simulink model "DC_Motor_Modelling"  (R2022b)
settings: Solver=VariableStepAuto  StartTime=0.0  StopTime=100.0  RelTol=1e-3
undefined symbols (not defined in the file): J, Kb, Ktq, L, plecs, R
libraries: ee_lib x3, fl_lib x1
settings Model: Creator=tedro  LastModifiedBy=tedro

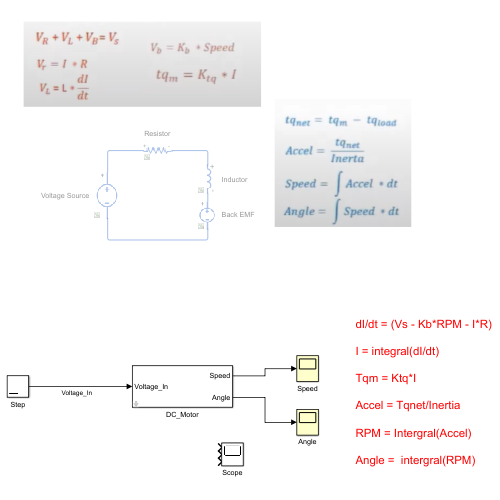
[thumbnail: Simulink's stored preview of the top-level diagram]
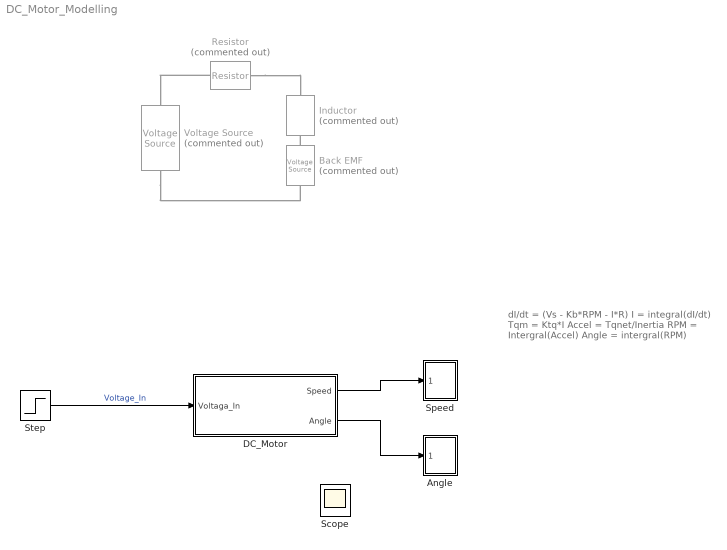
== system DC_Motor_Modelling ==
  note: dI/dt = (Vs - Kb*RPM - I*R)
      |
      | I = integral(dI/dt)
      |
      | Tqm = Ktq*I
      |
      | Accel = Tqnet/Inertia
      |
      | RPM = Intergral(Accel)
      |
      | Angle = intergral(RPM)
  Angle : Subsystem  LoadFcn=plecs('sl', 300);  InitFcn=plecs('sl', 314);  StartFcn=plecs('sl', 308);  StopFcn=plecs('sl', 309);  mask{Settings=<binary blob, 1052 chars, not shown>}
      mask init:
      | plecs('sl', 315);
      settings: CopyFcn=plecs('sl', 303);  DeleteFcn=plecs('sl', 305);  UndoDeleteFcn=plecs('sl', 306);  PreSaveFcn=plecs('sl', 311);  NameChangeFcn=plecs('sl', 310);  DestroyFcn=plecs('sl', 307);  OpenFcn=plecs('sl', 302);  ErrorFcn=plerrorfcn
      mask Display: plot([0.1 0.9 0.9 0.1 0.1], [0.9 0.9 0.5 0.5 0.9])
  Back EMF : ee_lib/Sources/Voltage Source  Commented=on  dc_voltage=0 V  ac_voltage=0 V  ac_shift=0 rad  ac_frequency=60 Hz  noise_mode=ee.enum.sources.noise.Disabled  PSD=0 V^2/Hz  sample_time=1e-3 s  repeatability=ee.enum.sources.repeatability.NotRepeatable  user_seed=0  auto_seed=3890346746  i_specify=off  i_priority=None  i=0 A  i_nominal_specify=off  i_nominal_unit=A  i_nominal_value=1  v_specify=off  v_priority=None  v=0 V  v_nominal_specify=off  v_nominal_unit=V  v_nominal_value=1
  DC_Motor : Subsystem
      mask Display:
      | port_label('input', 1, 'Voltage_In');
      | port_label('output', 1, 'Speed');
      | port_label('output', 2, 'Angle');
  Inductor : ee_lib/Passive/Inductor  Commented=on  l=1e-6 H  enable_L_tol=0  L_tol=20  tol_distribution=1  nSigma=4  r=0 Ohm  g=1e-9 1/Ohm  enable_operating_limits=0  operating_limit_action=2  max_working_current=1 A  power_rating=1 W  enable_faults=0  fault_action=1  lambdaPercent=50  k_faulted=0.9999  turnsShort=0  openCct=0  groundShort=0  groundShortG=0 1/Ohm  tau_fault=1e-3 s  enable_temporal_fault=0  t_fault=1 s  enable_behavioral_fault=0  max_permissible_voltage=100 V  n_fail_on_voltage=1  max_permissible_current=1 A  t_fail_on_current=1 s  i_L_specify=off  i_L_priority=High  i_L=0 A  i_L_nominal_specify=off  i_L_nominal_unit=A  i_L_nominal_value=1
  Resistor : fl_lib/Electrical/Electrical Elements/Resistor  Commented=on  R=1 Ohm  i_specify=off  i_priority=None  i=0 A  i_nominal_specify=off  i_nominal_unit=A  i_nominal_value=1  v_specify=off  v_priority=None  v=0 V  v_nominal_specify=off  v_nominal_unit=V  v_nominal_value=1
  Scope : Scope  NumInputPorts=3
  Speed : Subsystem  LoadFcn=plecs('sl', 300);  InitFcn=plecs('sl', 314);  StartFcn=plecs('sl', 308);  StopFcn=plecs('sl', 309);  mask{Settings=<binary blob, 1032 chars, not shown>}
      mask init:
      | plecs('sl', 315);
      settings: CopyFcn=plecs('sl', 303);  DeleteFcn=plecs('sl', 305);  UndoDeleteFcn=plecs('sl', 306);  PreSaveFcn=plecs('sl', 311);  NameChangeFcn=plecs('sl', 310);  DestroyFcn=plecs('sl', 307);  OpenFcn=plecs('sl', 302);  ErrorFcn=plerrorfcn
      mask Display: plot([0.1 0.9 0.9 0.1 0.1], [0.9 0.9 0.5 0.5 0.9])
  Step : Step  After=12  SampleTime=0
  Voltage Source : ee_lib/Sources/Voltage Source  Commented=on  dc_voltage=0 V  ac_voltage=0 V  ac_shift=0 rad  ac_frequency=60 Hz  noise_mode=ee.enum.sources.noise.Disabled  PSD=0 V^2/Hz  sample_time=1e-3 s  repeatability=ee.enum.sources.repeatability.NotRepeatable  user_seed=0  auto_seed=3499211588  i_specify=off  i_priority=None  i=0 A  i_nominal_specify=off  i_nominal_unit=A  i_nominal_value=1  v_specify=off  v_priority=None  v=0 V  v_nominal_specify=off  v_nominal_unit=V  v_nominal_value=1
  wires:
  Step/1 -> DC_Motor/1(Voltaga_In)  "Voltage_In"
  DC_Motor/2(Angle) -> Angle/1(1)
  DC_Motor/1(Speed) -> Speed/1(1)
  connections:
  Resistor/LConn1 -- Voltage Source/LConn1
  Resistor/RConn1 -- Inductor/LConn1
  Back EMF/LConn1 -- Inductor/RConn1
  Voltage Source/RConn1 -- Back EMF/RConn1

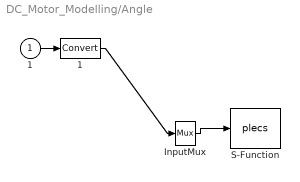
== system DC_Motor_Modelling/Angle ==
  1 : Inport
  " 1 " : DataTypeConversion
  " InputMux " : Mux  Inputs=1
  " S-Function " : S-Function  FunctionName=plecs  SFunctionDeploymentMode=off  EnableBusSupport=off
  wires:
  " InputMux "/1 -> " S-Function "/1
  1/1 -> " 1 "/1
  " 1 "/1 -> " InputMux "/1

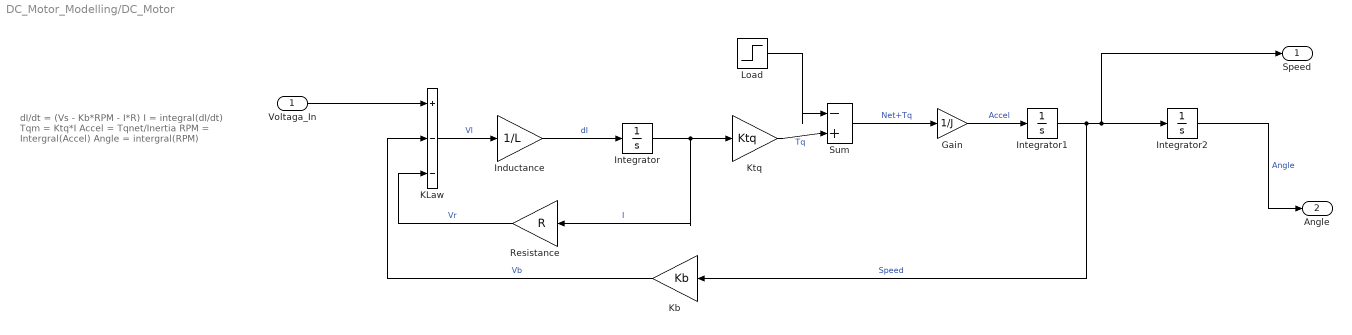
== system DC_Motor_Modelling/DC_Motor ==
  note: dI/dt = (Vs - Kb*RPM - I*R)
      |
      | I = integral(dI/dt)
      |
      | Tqm = Ktq*I
      |
      | Accel = Tqnet/Inertia
      |
      | RPM = Intergral(Accel)
      |
      | Angle = intergral(RPM)
  Voltaga_In : Inport
  Gain : Gain  Gain=1/J
  Inductance : Gain  Gain=1/L
  Integrator : Integrator
  Integrator1 : Integrator
  Integrator2 : Integrator
  KLaw : Sum  Inputs=+--
  Kb : Gain  Gain=Kb
  Ktq : Gain  Gain=Ktq
  Load : Step  Time=50  After=200  SampleTime=0
  Resistance : Gain  Gain=R
  Sum : Sum  Inputs=|-+
  Speed : Outport
  Angle : Outport  Port=2
  wires:
  Voltaga_In/1 -> KLaw/1
  KLaw/1 -> Inductance/1  "Vl"
  Inductance/1 -> Integrator/1  "dI"
  Integrator/1 -> Ktq/1, Resistance/1  "I"
  Resistance/1 -> KLaw/3  "Vr"
  Load/1 -> Sum/1
  Ktq/1 -> Sum/2  "Tq"
  Sum/1 -> Gain/1  "Net+Tq"
  Gain/1 -> Integrator1/1  "Accel"
  Integrator1/1 -> Speed/1, Integrator2/1, Kb/1  "Speed"
  Kb/1 -> KLaw/2  "Vb"
  Integrator2/1 -> Angle/1  "Angle"

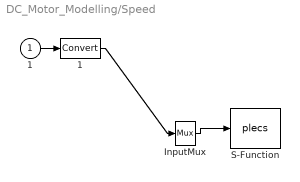
== system DC_Motor_Modelling/Speed ==
  1 : Inport
  " 1 " : DataTypeConversion
  " InputMux " : Mux  Inputs=1
  " S-Function " : S-Function  FunctionName=plecs  SFunctionDeploymentMode=off  EnableBusSupport=off
  wires:
  " InputMux "/1 -> " S-Function "/1
  1/1 -> " 1 "/1
  " 1 "/1 -> " InputMux "/1
